simulink model "transmitter"  (R2020b)
settings: Solver=FixedStepDiscrete  StartTime=0.0  StopTime=100000  RelTol=1e-3
undefined symbols (not defined in the file): message
libraries: hdlsllib x24, simulink x11, dspmlti4 x2, whdlio x1
(part 1 of 2)
settings Model: DataTypeOverride=Off  Creator=wardo  LastModifiedBy=wardo
settings DataIOCC: LimitDataPoints=on  SaveOutput=off  SaveTime=off
settings OptimizationCC: BlockReduction=off  ConditionallyExecuteInputs=off  DefaultParameterBehavior=Inlined  LifeSpan=inf
settings DebuggingCC: AlgebraicLoopMsg=error  SingleTaskRateTransMsg=error  AllowSymbolicDim=off  StrictBusMsg=ErrorOnBusTreatedAsVector  SFUnexpectedBacktrackingDiag=warning  SFNoUnconditionalDefaultTransitionDiag=warning  SFExecutionAtInitializationDiag=none  ArithmeticOperatorsInVariantConditions=warning
settings HardwareCC: ProdBitPerPointer=32  ProdBitPerSizeT=32  ProdBitPerPtrDiffT=32  ProdLargestAtomicFloat=None  ProdIntDivRoundTo=Undefined  ProdEndianess=Unspecified  ProdWordSize=32  ProdHWDeviceType=ASIC/FPGA->ASIC/FPGA  ProdEqTarget=off
settings SFSimCC: SimUseLocalCustomCode=off  CustomCodeUndefinedFunction=UseInterfaceOnly
settings RTWCC: RTWUseLocalCustomCode=off
settings CodeAppCC: StateflowObjectComments=on
settings GRTTargetCC: TargetLangStandard=C89/C90 (ANSI)
settings ConfigComp: CovScope=ReferencedModels  CovMetricSettings=dw  CovSaveCumulativeToWorkspaceVar=on  CovSaveSingleToWorkspaceVar=on  CovExternalEMLEnable=off  CovSFcnEnable=off

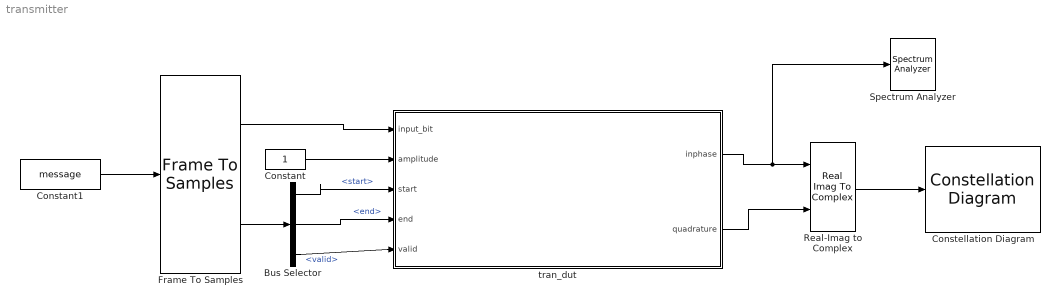
== system transmitter ==
  Bus Selector : BusSelector  OutputSignals=start,end,valid
  Constant : Constant  OutDataTypeStr=uint8  SampleTime=-1
  Constant1 : Constant  Value=message  OutDataTypeStr=fixdt(0,1,0)  SampleTime=100000
  Constellation Diagram : ConstellationDiagram
  Frame To Samples : whdlio/Frame To Samples  InterSampleIdleCycles=0  InterFrameIdleCycles=0  OutputSize=1  InterleaveSamples=off
      settings: SourceProductBaseCode=LH
  Real-Imag to Complex : RealImagToComplex
  Spectrum Analyzer : SpectrumAnalyzer
  tran_dut : Subsystem
  wires:
  Frame To Samples/1 -> tran_dut/1(input_bit)
  Constant/1 -> tran_dut/2(amplitude)
  Constant1/1 -> Frame To Samples/1
  Real-Imag to Complex/1 -> Constellation Diagram/1
  tran_dut/1(inphase) -> Spectrum Analyzer/1, Real-Imag to Complex/1
  tran_dut/2(quadrature) -> Real-Imag to Complex/2
  Frame To Samples/2 -> Bus Selector/1
  Bus Selector/1 -> tran_dut/3(start)  "<start>"
  Bus Selector/2 -> tran_dut/4(end)  "<end>"
  Bus Selector/3 -> tran_dut/5(valid)  "<valid>"

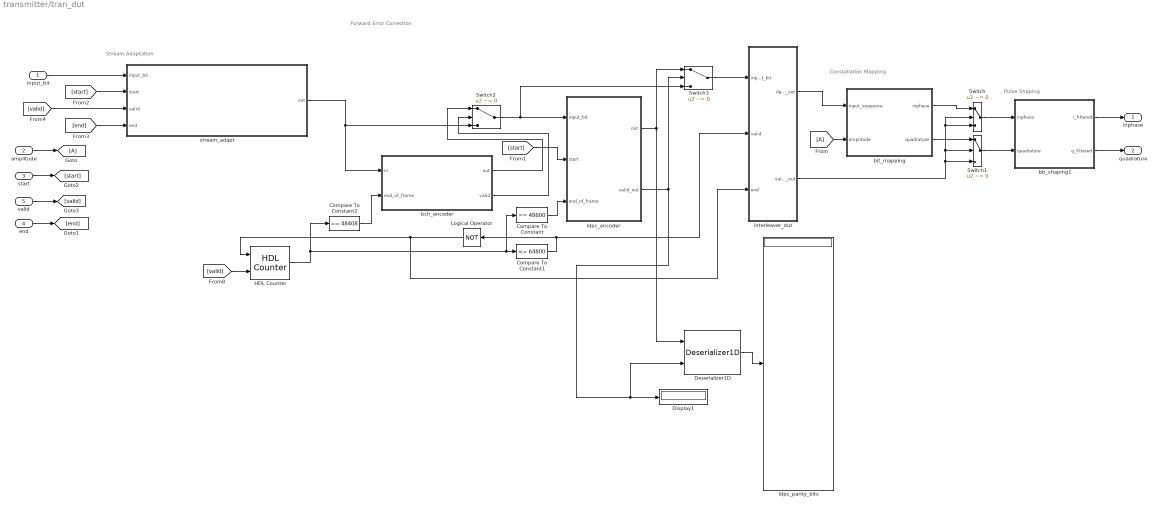
== system transmitter/tran_dut ==
  note: Pulse Shaping
  note: Constellation Mapping
  note: Forward Error Correction
  note: Stream Adaptation
  input_bit : Inport
  amplitude : Inport  Port=2
  start : Inport  Port=3
  end : Inport  Port=4
  valid : Inport  Port=5
  Compare To Constant : simulink/Logic and Bit Operations/Compare To Constant  relop===  const=48600  OutDataTypeStr=boolean
  Compare To Constant1 : simulink/Logic and Bit Operations/Compare To Constant  relop=<=  const=64800  OutDataTypeStr=boolean
  Compare To Constant2 : simulink/Logic and Bit Operations/Compare To Constant  relop===  const=48408  OutDataTypeStr=boolean
  Deserializer1D : hdlsllib/HDL Operations/Deserializer1D  Ratio=16200  IdleCycles=0  InitialCondition=0  startIn=off  validIn=on  validOut=off  inputDataDimensions=-1  inputSampleTime=-1  inputSignalType=auto
      settings: SourceProductBaseCode=SL
  Display1 : Display
  HDL Counter : hdlsllib/Sources/HDL Counter  CountType=Count limited  CountInit=0  CountStep=1  CountMax=64800  CountFromType=Initial value  CountFrom=0  CountResetPort=on  CountLoadPort=off  CountEnbPort=on  CountDirPort=off  CountDataType=Unsigned  CountWordLen=16  CountFracLen=0  CountSampTime=1
  Logical Operator : Logic  Operator=NOT  IconShape=distinctive  AllPortsSameDT=off  OutDataTypeStr=boolean
  Switch : Switch  Criteria=u2 ~= 0  OutDataTypeStr=Inherit: Inherit via back propagation
  Switch1 : Switch  Criteria=u2 ~= 0  OutDataTypeStr=Inherit: Inherit via back propagation
  Switch2 : Switch  Criteria=u2 ~= 0  OutDataTypeStr=boolean
  Switch3 : Switch  Criteria=u2 ~= 0  OutDataTypeStr=boolean
  bb_shaping1 : Subsystem
  bch_encoder : Subsystem
  bit_mapping : Subsystem
  interleaver_dut : Subsystem
  ldpc_encoder : Subsystem
  ldpc_parity_bits : Display
  stream_adapt : Subsystem
  inphase : Outport  VectorParamsAs1DForOutWhenUnconnected=off
  quadrature : Outport  Port=2  VectorParamsAs1DForOutWhenUnconnected=off
  wires:
  bb_shaping1/1(i_filtered) -> inphase/1
  bb_shaping1/2(q_filtered) -> quadrature/1
  bit_mapping/2(quadrature) -> Switch1/1
  bit_mapping/1(inphase) -> Switch/1
  interleaver_dut/2(valid_out) -> Switch1/2, Switch/2, Switch/3, Switch1/3
  Switch/1 -> bb_shaping1/1(inphase)
  Switch1/1 -> bb_shaping1/2(quadrature)
  ldpc_encoder/1(out) -> Deserializer1D/1, Switch3/1
  Deserializer1D/1 -> ldpc_parity_bits/1
  ldpc_encoder/2(valid_out) -> Deserializer1D/2, Display1/1, Switch3/2
  stream_adapt/1(out) -> Switch2/3, bch_encoder/1(in)
  Switch2/1 -> ldpc_encoder/1(input_bit), Switch3/3
  bch_encoder/2(valid) -> Switch2/2
  amplitude/1 -> [A]
  [A] -> bit_mapping/2(amplitude)
  end/1 -> [end]
  bch_encoder/1(out) -> Switch2/1
  start/1 -> [start]
  [start] -> stream_adapt/2(start)
  input_bit/1 -> stream_adapt/1(input_bit)
  [end] -> stream_adapt/4(end)
  valid/1 -> [valid]
  [valid] -> stream_adapt/3(valid)
  Compare To Constant2/1 -> bch_encoder/2(end_of_frame)
  Switch3/1 -> interleaver_dut/1(input_bit)
  [start] -> ldpc_encoder/2(start)
  HDL Counter/1 -> Compare To Constant2/1, Compare To Constant/1, Compare To Constant1/1
  Compare To Constant/1 -> ldpc_encoder/3(end_of_frame)
  [valid] -> HDL Counter/2
  Compare To Constant1/1 -> interleaver_dut/2(valid), Logical Operator/1
  Logical Operator/1 -> interleaver_dut/3(end), HDL Counter/1
  interleaver_dut/1(data_out) -> bit_mapping/1(input_sequence)

== system transmitter/tran_dut/bb_shaping1 ==
  inphase : Inport
  quadrature : Inport  Port=2
  FIR Interpolation : dspmlti4/FIR Interpolation  FilterSource=Dialog parameters  PrivateCoeffs=0  h=[-0.00599670410156250,-0.00514221191406250,-0.00289916992187500,0.000442504882812500,0.00431823730468750,0.00794982910156250,0.0104980468750000,0.0112304687500000,0.00967407226562500,0.00578308105468750,0,-0.00680541992187500,-0.0134124755859375,-0.0184326171875000,-0.0205841064453125,-0.0189819335937500,-0.0133361816406250,-0.00410461425781250,0.00752258300781250,0.0196380615234375,0.0300140380859375,0.0363464355468750,0.0367584228515625,0.0301208496093750,0.0164794921875000,-0.00291442871093750,-0.0254821777343750,-0.0476837158203125,-0.0653228759765625,-0.0742187500000000,-0.0707244873046875,-0.0524291992187500,-0.0185852050781250,0.0296783447265625,0.0892028808593750,0.155227661132813,0.221755981445313,0.282333374023438,0.330810546875000,0.362121582031250,0.372940063476563,0.362121582031250,0.330810546875000,0.282333374023438,0.221755981445313,0.155227661132813,0.0892028808593750,0.0296783447265625,-0.0185852050781250,-0.0524291992187500,-0.0707244873046875,-0.0742187500000000,-0.0653228759765625,-0.0476837158203125,-0.0254821777343750,-0.00291442871093750,0.0164794921875000,0.0301208496093750,0.0367584228515625,0.0363464355468750,0.0300140380859375,0.0196380615234375,0.00752258300781250,-0.00410461425781250,-0.0133361816406250,-0.0189819335937500,-0.0205841064453125,-0.0184326171875000,-0.0134124755859375,-0.00680541992187500,0,0.00578308105468750,0.00967407226562500,0.0112304687500000,0.0104980468750000,0.00794982910156250,0.00431823730468750,0.000442504882812500,-0.00289916992187500,-0.00514221191406250,-0.00599670410156250]  L=8  FilterObject=FINTERP  framing=Allow multirate processing  outputBufInitCond=0  roundingMode=Floor  overflowMode=off  firstCoeffMode=Specify word length  firstCoeffWordLength=16  firstCoeffFracLength=15  firstCoeffDataTypeStr=fixdt(1,16)  firstCoeffMin=[]  firstCoeffMax=[]  firstCoeffLastDataTypeStr=fixdt(1,16)  outputDataTypeStr=Inherit: Same as accumulator  outputMin=[]  outputMax=[]  outputLastDataTypeStr=Inherit: Same as accumulator
      settings: SourceProductName=DSP System Toolbox
  FIR Interpolation1 : dspmlti4/FIR Interpolation  FilterSource=Dialog parameters  PrivateCoeffs=0  h=[-0.00599670410156250,-0.00514221191406250,-0.00289916992187500,0.000442504882812500,0.00431823730468750,0.00794982910156250,0.0104980468750000,0.0112304687500000,0.00967407226562500,0.00578308105468750,0,-0.00680541992187500,-0.0134124755859375,-0.0184326171875000,-0.0205841064453125,-0.0189819335937500,-0.0133361816406250,-0.00410461425781250,0.00752258300781250,0.0196380615234375,0.0300140380859375,0.0363464355468750,0.0367584228515625,0.0301208496093750,0.0164794921875000,-0.00291442871093750,-0.0254821777343750,-0.0476837158203125,-0.0653228759765625,-0.0742187500000000,-0.0707244873046875,-0.0524291992187500,-0.0185852050781250,0.0296783447265625,0.0892028808593750,0.155227661132813,0.221755981445313,0.282333374023438,0.330810546875000,0.362121582031250,0.372940063476563,0.362121582031250,0.330810546875000,0.282333374023438,0.221755981445313,0.155227661132813,0.0892028808593750,0.0296783447265625,-0.0185852050781250,-0.0524291992187500,-0.0707244873046875,-0.0742187500000000,-0.0653228759765625,-0.0476837158203125,-0.0254821777343750,-0.00291442871093750,0.0164794921875000,0.0301208496093750,0.0367584228515625,0.0363464355468750,0.0300140380859375,0.0196380615234375,0.00752258300781250,-0.00410461425781250,-0.0133361816406250,-0.0189819335937500,-0.0205841064453125,-0.0184326171875000,-0.0134124755859375,-0.00680541992187500,0,0.00578308105468750,0.00967407226562500,0.0112304687500000,0.0104980468750000,0.00794982910156250,0.00431823730468750,0.000442504882812500,-0.00289916992187500,-0.00514221191406250,-0.00599670410156250]  L=8  FilterObject=FINTERP  framing=Allow multirate processing  outputBufInitCond=0  roundingMode=Floor  overflowMode=off  firstCoeffMode=Specify word length  firstCoeffWordLength=16  firstCoeffFracLength=15  firstCoeffDataTypeStr=fixdt(1,16)  firstCoeffMin=[]  firstCoeffMax=[]  firstCoeffLastDataTypeStr=fixdt(1,16)  outputDataTypeStr=Inherit: Same as accumulator  outputMin=[]  outputMax=[]  outputLastDataTypeStr=Inherit: Same as accumulator
      settings: SourceProductName=DSP System Toolbox
  i_filtered : Outport  VectorParamsAs1DForOutWhenUnconnected=off
  q_filtered : Outport  Port=2  VectorParamsAs1DForOutWhenUnconnected=off
  wires:
  inphase/1 -> FIR Interpolation/1
  FIR Interpolation/1 -> i_filtered/1
  FIR Interpolation1/1 -> q_filtered/1
  quadrature/1 -> FIR Interpolation1/1

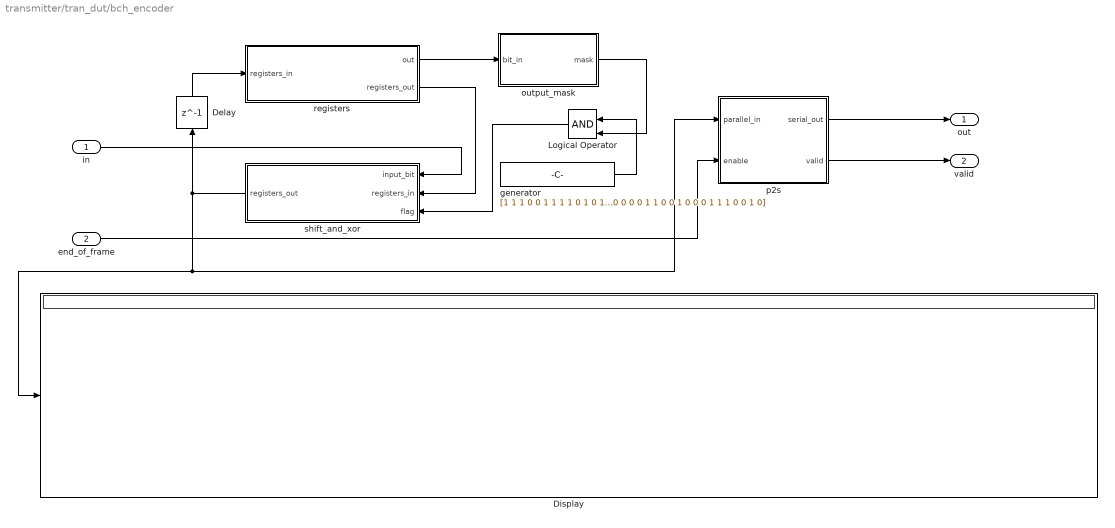
== system transmitter/tran_dut/bch_encoder ==
  in : Inport
  end_of_frame : Inport  Port=2
  Delay : Delay  DelayLength=1
  Display : Display
  Logical Operator : Logic  IconShape=distinctive  AllPortsSameDT=off  OutDataTypeStr=fixdt(0, 1, 0)
  generator : Constant  Value=|  OutDataTypeStr=fixdt(0, 1, 0)  SampleTime=-1
      | [1
      | 1
      | 1
      | 0
      | 0
      | 1
      | 1
      | 1
      | 1
      | 0
      | 1
      | 0
      | 1
      | 0
      | 1
      | 0
      | 0
      | 1
      | 0
      | 0
      | 0
      | 0
      | 0
      | 0
      | 0
      | 1
      | 1
      | 0
      | 0
      | 1
      | 1
      | 0
      | 1
      | 1
      | 1
      | 0
      | 1
      | 1
      | 1
      | 1
      | 1
      | 0
      | 1
      | 0
      | 0
      | 0
      | 0
      | 1
      | 1
      | 1
      | 1
      | 0
      | 0
      | 0
      | 1
      | 0
      | 1
      | 1
      | 0
      | 0
      | 0
      | 0
      | 0
      | 0
      | 1
      | 0
      | 0
      | 1
      | 0
      | 0
      | 0
      | 1
      | 0
      | 0
      | 0
      | 1
      | 0
      | 0
      | 0
      | 0
      | 1
      | 0
      | 1
      | 0
      | 1
      | 1
      | 0
      | 0
      | 0
      | 0
      | 1
      | 1
      | 1
      | 0
      | 1
      | 1
      | 0
      | 0
      | 0
      | 1
      | 1
      | 0
      | 1
      | 1
      | 0
      | 0
      | 1
      | 1
      | 0
      | 1
      | 0
      | 0
      | 1
      | 1
      | 1
      | 1
      | 0
      | 0
      | 1
      | 1
      | 0
      | 0
      | 0
      | 0
      | 1
      | 0
      | 1
      | 0
      | 0
      | 0
      | 1
      | 1
      | 1
      | 0
      | 0
      | 0
      | 1
      | 0
      | 0
      | 0
      | 1
      | 0
      | 1
      | 0
      | 0
      | 0
      | 1
      | 1
      | 1
      | 0
      | 1
      | 0
      | 0
      | 0
      | 1
      | 0
      | 0
      | 0
      | 0
      | 1
      | 1
      | 1
      | 0
      | 0
      | 0
      | 0
      | 0
      | 1
      | 0
      | 1
      | 1
      | 1
      | 0
      | 0
      | 0
      | 0
      | 0
      | 1
      | 1
      | 0
      | 0
      | 1
      | 0
      | 0
      | 0
      | 1
      | 1
      | 1
      | 0
      | 0
      | 1
      | 0]
  output_mask : MATLAB Function  TreatAsAtomicUnit=on
  p2s : MATLAB Function  TreatAsAtomicUnit=on  mask{input_length=192}
  registers : MATLAB Function  TreatAsAtomicUnit=on
  shift_and_xor : MATLAB Function  TreatAsAtomicUnit=on
  out : Outport  VectorParamsAs1DForOutWhenUnconnected=off
  valid : Outport  Port=2  VectorParamsAs1DForOutWhenUnconnected=off
  wires:
  registers/1(out) -> output_mask/1(bit_in)
  output_mask/1(mask) -> Logical Operator/2
  generator/1 -> Logical Operator/1
  Logical Operator/1 -> shift_and_xor/3(flag)
  registers/2(registers_out) -> shift_and_xor/2(registers_in)
  shift_and_xor/1(registers_out) -> p2s/1(parallel_in), Display/1, Delay/1
  in/1 -> shift_and_xor/1(input_bit)
  Delay/1 -> registers/1(registers_in)
  end_of_frame/1 -> p2s/2(enable)
  p2s/1(serial_out) -> out/1
  p2s/2(valid) -> valid/1

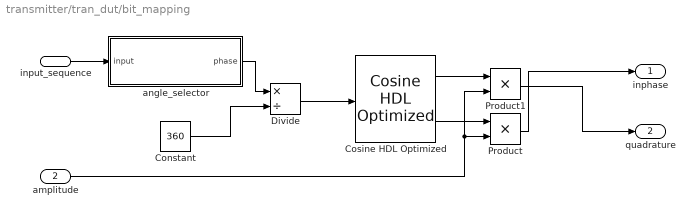
== system transmitter/tran_dut/bit_mapping ==
  input_sequence : Inport
  amplitude : Inport  Port=2
  Constant : Constant  Value=360  OutDataTypeStr=fixdt(0,9,0)  SampleTime=-1
  Cosine HDL Optimized : hdlsllib/Lookup Tables/Cosine HDL Optimized  OutputFormula=sin(2*pi*u) and cos(2*pi*u)  NumDataPoints=32  TableDataTypeStr=fixdt(1,16,15)  SimulateLUTROMDelay=off
      settings: SourceProductBaseCode=SL
  Divide : Product  Inputs=*/  OutMin=0  OutMax=1  OutDataTypeStr=fixdt(1,16,14)  RndMeth=Zero  SaturateOnIntegerOverflow=on
  Product : Product
  Product1 : Product
  angle_selector : MATLAB Function  TreatAsAtomicUnit=on
  inphase : Outport  VectorParamsAs1DForOutWhenUnconnected=off
  quadrature : Outport  Port=2  VectorParamsAs1DForOutWhenUnconnected=off
  wires:
  Product/1 -> inphase/1
  Product1/1 -> quadrature/1
  input_sequence/1 -> angle_selector/1(input)
  amplitude/1 -> Product1/2, Product/2
  Cosine HDL Optimized/2 -> Product/1
  Cosine HDL Optimized/1 -> Product1/1
  Divide/1 -> Cosine HDL Optimized/1
  angle_selector/1(phase) -> Divide/1
  Constant/1 -> Divide/2

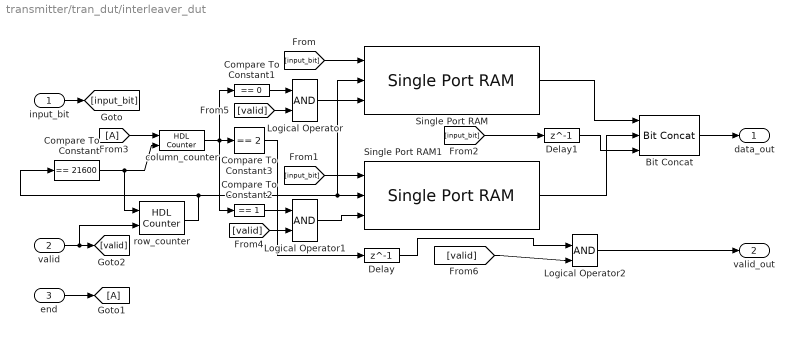
== system transmitter/tran_dut/interleaver_dut ==
  input_bit : Inport
  valid : Inport  Port=2
  end : Inport  Port=3
  Bit Concat : hdlsllib/Logic and Bit Operations/Bit Concat  numInputs=3
  Compare To Constant : simulink/Logic and Bit Operations/Compare To Constant  relop===  const=21600  OutDataTypeStr=boolean
  Compare To Constant1 : simulink/Logic and Bit Operations/Compare To Constant  relop===  const=0  OutDataTypeStr=boolean
  Compare To Constant2 : simulink/Logic and Bit Operations/Compare To Constant  relop===  const=1  OutDataTypeStr=boolean
  Compare To Constant3 : simulink/Logic and Bit Operations/Compare To Constant  relop===  const=2  OutDataTypeStr=boolean
  Delay : Delay  DelayLength=1
  Delay1 : Delay  DelayLength=1
  Logical Operator : Logic  IconShape=distinctive  AllPortsSameDT=off  OutDataTypeStr=boolean
  Logical Operator1 : Logic  IconShape=distinctive  AllPortsSameDT=off  OutDataTypeStr=boolean
  Logical Operator2 : Logic  IconShape=distinctive  AllPortsSameDT=off  OutDataTypeStr=boolean
  Single Port RAM : hdlsllib/HDL RAMs/Single Port RAM  ram_size=15  dout_type=New data
      settings: SourceProductBaseCode=SL
  Single Port RAM1 : hdlsllib/HDL RAMs/Single Port RAM  ram_size=15  dout_type=New data
      settings: SourceProductBaseCode=SL
  column_counter : hdlsllib/Sources/HDL Counter  CountType=Count limited  CountInit=0  CountStep=1  CountMax=2  CountFromType=Initial value  CountFrom=0  CountResetPort=on  CountLoadPort=off  CountEnbPort=on  CountDirPort=off  CountDataType=Unsigned  CountWordLen=3  CountFracLen=0  CountSampTime=1
  row_counter : hdlsllib/Sources/HDL Counter  CountType=Count limited  CountInit=1  CountStep=1  CountMax=21600  CountFromType=Initial value  CountFrom=1  CountResetPort=on  CountLoadPort=off  CountEnbPort=on  CountDirPort=off  CountDataType=Unsigned  CountWordLen=15  CountFracLen=0  CountSampTime=1
  data_out : Outport  VectorParamsAs1DForOutWhenUnconnected=off
  valid_out : Outport  Port=2  VectorParamsAs1DForOutWhenUnconnected=off
  wires:
  Bit Concat/1 -> data_out/1
  Logical Operator2/1 -> valid_out/1
  row_counter/1 -> Single Port RAM/2, Single Port RAM1/2, Compare To Constant/1
  Compare To Constant/1 -> column_counter/2, row_counter/1
  input_bit/1 -> [input_bit]
  [input_bit] -> Single Port RAM/1
  [input_bit] -> Single Port RAM1/1
  Compare To Constant1/1 -> Logical Operator/1
  column_counter/1 -> Compare To Constant1/1, Compare To Constant3/1, Compare To Constant2/1
  Logical Operator/1 -> Single Port RAM/3
  Logical Operator1/1 -> Single Port RAM1/3
  Compare To Constant2/1 -> Logical Operator1/1
  Single Port RAM1/1 -> Bit Concat/2
  Single Port RAM/1 -> Bit Concat/1
  Compare To Constant3/1 -> Delay/1
  [input_bit] -> Delay1/1
  end/1 -> [A]
  [A] -> column_counter/1
  valid/1 -> row_counter/2, [valid]
  [valid] -> Logical Operator2/2
  [valid] -> Logical Operator/2
  [valid] -> Logical Operator1/2
  Delay/1 -> Logical Operator2/1
  Delay1/1 -> Bit Concat/3

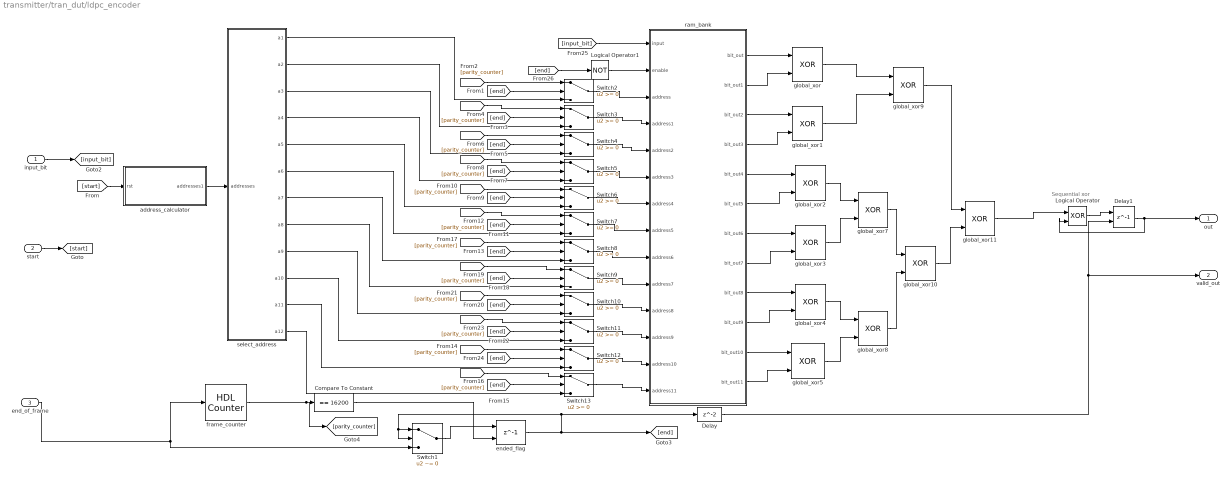
== system transmitter/tran_dut/ldpc_encoder ==
  note: Sequential xor
  input_bit : Inport
  start : Inport  Port=2
  end_of_frame : Inport  Port=3
  Compare To Constant : simulink/Logic and Bit Operations/Compare To Constant  relop===  const=16200  OutDataTypeStr=boolean
  Delay : Delay
  Delay1 : Delay  DelayLength=1  ShowEnablePort=on
      settings: InputPortMap=u0,e6
  Logical Operator : Logic  Operator=XOR  IconShape=distinctive  AllPortsSameDT=off  OutDataTypeStr=fixdt(0,1, 0)
  Logical Operator1 : Logic  Operator=NOT  IconShape=distinctive  AllPortsSameDT=off  OutDataTypeStr=boolean
  Switch1 : Switch  Criteria=u2 ~= 0  OutDataTypeStr=boolean
  Switch{2..13} (12 alike) : Switch
  address_calculator : Subsystem
  ended_flag : Delay  DelayLength=1  ExternalReset=Level
      settings: InputPortMap=u0,r5
  frame_counter : hdlsllib/Sources/HDL Counter  CountType=Count limited  CountInit=0  CountStep=1  CountMax=16200  CountFromType=Initial value  CountFrom=0  CountResetPort=on  CountLoadPort=off  CountEnbPort=off  CountDirPort=off  CountDataType=Unsigned  CountWordLen=14  CountFracLen=0  CountSampTime=1
  global_xor{,1..5,7..11} (11 alike) : Logic  Operator=XOR  IconShape=distinctive  AllPortsSameDT=off  OutDataTypeStr=boolean
  ram_bank : Subsystem
  select_address : MATLAB Function  TreatAsAtomicUnit=on
  out : Outport  VectorParamsAs1DForOutWhenUnconnected=off
  valid_out : Outport  Port=2  VectorParamsAs1DForOutWhenUnconnected=off
  wires:
  input_bit/1 -> [input_bit]
  start/1 -> [start]
  address_calculator/1(addresses1) -> select_address/1(addresses)
  [start] -> address_calculator/1(rst)
  Logical Operator/1 -> Delay1/1
  Delay1/1 -> out/1, Logical Operator/2
  Compare To Constant/1 -> ended_flag/2
  Switch1/1 -> ended_flag/1
  frame_counter/1 -> [parity_counter], Compare To Constant/1
  ram_bank/1(bit_out) -> global_xor/1
  [end] -> Switch2/2
  select_address/1(a1) -> Switch2/3
  [parity_counter] -> Switch2/1
  Switch3/1 -> ram_bank/4(address1)
  [parity_counter] -> Switch3/1
  [end] -> Switch3/2
  select_address/2(a2) -> Switch3/3
  [end] -> Switch5/2
  select_address/3(a3) -> Switch4/3
  [parity_counter] -> Switch5/1
  [end] -> Switch4/2
  select_address/4(a4) -> Switch5/3
  [parity_counter] -> Switch4/1
  [parity_counter] -> Switch7/1
  [end] -> Switch6/2
  [parity_counter] -> Switch6/1
  [end] -> Switch7/2
  select_address/5(a5) -> Switch6/3
  select_address/6(a6) -> Switch7/3
  [end] -> Switch10/2
  [end] -> Switch9/2
  [end] -> Switch11/2
  [parity_counter] -> Switch13/1
  select_address/10(a10) -> Switch11/3
  select_address/11(a11) -> Switch12/3
  [parity_counter] -> Switch11/1
  [end] -> Switch8/2
  [end] -> Switch13/2
  select_address/8(a8) -> Switch9/3
  select_address/9(a9) -> Switch10/3
  [end] -> Switch12/2
  select_address/12(a12) -> Switch13/3
  [parity_counter] -> Switch12/1
  [parity_counter] -> Switch10/1
  [parity_counter] -> Switch9/1
  select_address/7(a7) -> Switch8/3
  [parity_counter] -> Switch8/1
  [input_bit] -> ram_bank/1(input)
  Switch2/1 -> ram_bank/3(address)
  Logical Operator1/1 -> ram_bank/2(enable)
  ram_bank/2(bit_out1) -> global_xor/2
  ram_bank/3(bit_out2) -> global_xor1/1
  ram_bank/4(bit_out3) -> global_xor1/2
  ram_bank/6(bit_out5) -> global_xor2/2
  ram_bank/8(bit_out7) -> global_xor3/2
  ram_bank/9(bit_out8) -> global_xor4/1
  ram_bank/10(bit_out9) -> global_xor4/2
  ram_bank/11(bit_out10) -> global_xor5/1
  ram_bank/12(bit_out11) -> global_xor5/2
  Switch4/1 -> ram_bank/5(address2)
  Switch5/1 -> ram_bank/6(address3)
  Switch6/1 -> ram_bank/7(address4)
  Switch7/1 -> ram_bank/8(address5)
  Switch8/1 -> ram_bank/9(address6)
  Switch9/1 -> ram_bank/10(address7)
  Switch10/1 -> ram_bank/11(address8)
  Switch11/1 -> ram_bank/12(address9)
  Switch12/1 -> ram_bank/13(address10)
  Switch13/1 -> ram_bank/14(address11)
  ram_bank/7(bit_out6) -> global_xor3/1
  ram_bank/5(bit_out4) -> global_xor2/1
  global_xor11/1 -> Logical Operator/1
  global_xor9/1 -> global_xor11/1
  global_xor10/1 -> global_xor11/2
  global_xor8/1 -> global_xor10/2
  global_xor7/1 -> global_xor10/1
  global_xor/1 -> global_xor9/1
  global_xor1/1 -> global_xor9/2
  global_xor2/1 -> global_xor7/1
  global_xor3/1 -> global_xor7/2
  global_xor4/1 -> global_xor8/1
  global_xor5/1 -> global_xor8/2
  ended_flag/1 -> [end], Switch1/2, Switch1/1, Delay/1
  [end] -> Logical Operator1/1
  end_of_frame/1 -> frame_counter/1, Switch1/3
  Delay/1 -> valid_out/1, Delay1/2

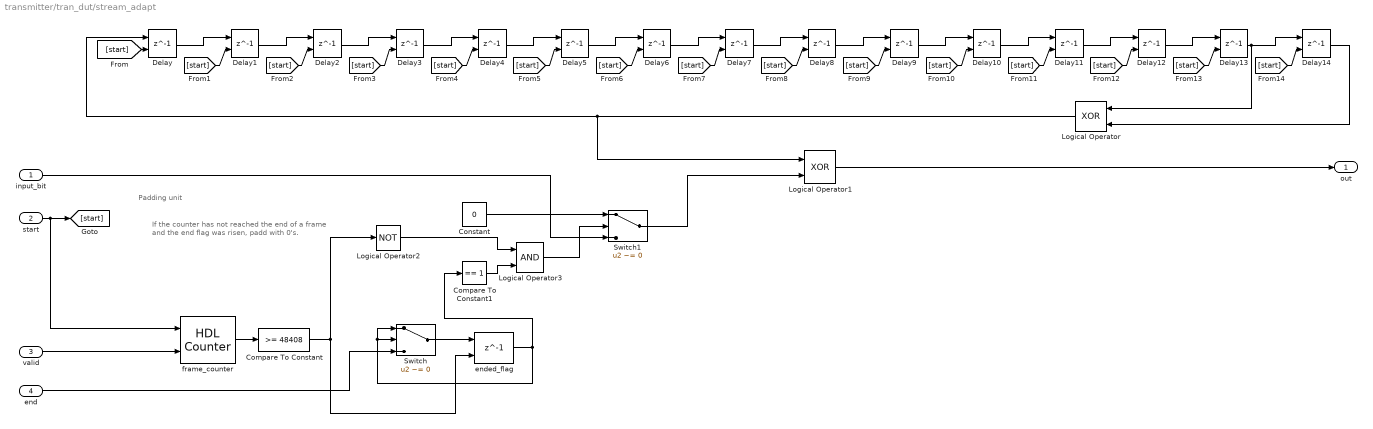
== system transmitter/tran_dut/stream_adapt ==
  note: Padding unit
  note: If the counter has not reached the end of a frame and the end flag was risen,
      | padd with 0's.
  input_bit : Inport
  start : Inport  Port=2
  valid : Inport  Port=3
  end : Inport  Port=4
  Compare To Constant : simulink/Logic and Bit Operations/Compare To Constant  relop=>=  const=48408  OutDataTypeStr=boolean
  Compare To Constant1 : simulink/Logic and Bit Operations/Compare To Constant  relop===  const=1  OutDataTypeStr=boolean
  Constant : Constant  Value=0  OutDataTypeStr=fixdt(0,1)  SampleTime=-1
  Delay{,3,5,7} (4 alike) : Delay  DelayLength=1  InitialCondition=1  ExternalReset=Level
      settings: InputPortMap=u0,r5
  Delay{1..2,4,6,8..14} (11 alike) : Delay  DelayLength=1  ExternalReset=Level
      settings: InputPortMap=u0,r5
  Logical Operator : Logic  Operator=XOR  IconShape=distinctive  AllPortsSameDT=off  OutDataTypeStr=boolean
  Logical Operator1 : Logic  Operator=XOR  IconShape=distinctive  AllPortsSameDT=off  OutDataTypeStr=boolean
  Logical Operator2 : Logic  Operator=NOT  IconShape=distinctive  AllPortsSameDT=off  OutDataTypeStr=boolean
  Logical Operator3 : Logic  IconShape=distinctive  AllPortsSameDT=off  OutDataTypeStr=boolean
  Switch : Switch  Criteria=u2 ~= 0  OutDataTypeStr=boolean
  Switch1 : Switch  Criteria=u2 ~= 0
  ended_flag : Delay  DelayLength=1  ExternalReset=Level
      settings: InputPortMap=u0,r5
  frame_counter : hdlsllib/Sources/HDL Counter  CountType=Count limited  CountInit=0  CountStep=1  CountMax=48408  CountFromType=Initial value  CountFrom=0  CountResetPort=on  CountLoadPort=off  CountEnbPort=on  CountDirPort=off  CountDataType=Unsigned  CountWordLen=16  CountFracLen=0  CountSampTime=1
  out : Outport  VectorParamsAs1DForOutWhenUnconnected=off
  wires:
  Delay/1 -> Delay1/1
  Logical Operator/1 -> Delay/1, Logical Operator1/1
  Logical Operator1/1 -> out/1
  start/1 -> frame_counter/1, [start]
  [start] -> Delay/2
  [start] -> Delay1/2
  Delay1/1 -> Delay2/1
  [start] -> Delay2/2
  Delay2/1 -> Delay3/1
  [start] -> Delay3/2
  Delay3/1 -> Delay4/1
  [start] -> Delay4/2
  Delay4/1 -> Delay5/1
  [start] -> Delay5/2
  Delay5/1 -> Delay6/1
  [start] -> Delay6/2
  Delay6/1 -> Delay7/1
  [start] -> Delay7/2
  Delay7/1 -> Delay8/1
  [start] -> Delay8/2
  Delay8/1 -> Delay9/1
  [start] -> Delay9/2
  Delay9/1 -> Delay10/1
  [start] -> Delay10/2
  Delay10/1 -> Delay11/1
  [start] -> Delay11/2
  Delay11/1 -> Delay12/1
  [start] -> Delay12/2
  Delay12/1 -> Delay13/1
  [start] -> Delay13/2
  Delay13/1 -> Logical Operator/1, Delay14/1
  [start] -> Delay14/2
  Delay14/1 -> Logical Operator/2
  valid/1 -> frame_counter/2
  frame_counter/1 -> Compare To Constant/1
  Compare To Constant/1 -> ended_flag/2, Logical Operator2/1
  Switch/1 -> ended_flag/1
  end/1 -> Switch/3
  ended_flag/1 -> Switch/1, Switch/2, Compare To Constant1/1
  Compare To Constant1/1 -> Logical Operator3/2
  Logical Operator3/1 -> Switch1/2
  Logical Operator2/1 -> Logical Operator3/1
  Switch1/1 -> Logical Operator1/2
  input_bit/1 -> Switch1/3
  Constant/1 -> Switch1/1

== system transmitter/tran_dut/ldpc_encoder/address_calculator ==
  rst : Inport
  addresses : MATLAB Function  TreatAsAtomicUnit=on  mask{bit_addresses=uint16([[0 6385 7901 14611 13389 11200 3252 5243 2504 2722 821 7374]; [1 11359 2698 357 13824 12772 7244 6752 15310 852 2001 11417]; [2 7862 7977 6321 13612 12197 14449 15137 13860 1708 6399 13444]; [3 1560 11804 6975 13292 3646 3812 8772 7306 5795 14327 7866]; [4 7626 11407 14599 9689 1628 2113 10809 9283 1230 15241 4870]; [5 1610 5699 15876 9446 12515 1400 6303 5411 14181 13925 7358]; [6 4059 8836 3405 7853 7992 15336 5970 10368 10278 9675 4651]; [7 4441 3963 9153 2109 12683 7459 12030 12221 629 15212 406]; [8 6007 8411 5771 3497 543 14202 875 9186 6235 13908 3563]; [9 3232 6625 4795 546 9781 2071 7312 3399 7250 4932 12652]; [10 8820 10088 11090 7069 6585 13134 10158 7183 488 7455 9238]; [11 1903 10818 119 215 7558 11046 10615 11545 14784 7961 15619]; [12 3655 8736 4917 15874 5129 2134 15944 14768 7150 2692 1469]; [13 8316 3820 505 8923 6757 806 7957 4216 15589 13244 2622]; [14 14463 4852 15733 3041 11193 12860 13673 8152 6551 15108 8758]; [15 3149 11981 16200 16200 16200 16200 16200 16200 16200 16200 16200]; [16 13416 6906 16200 16200 16200 16200 16200 16200 16200 16200 16200]; [17 13098 13352 16200 16200 16200 16200 16200 16200 16200 16200 16200]; [18 2009 14460 16200 16200 16200 16200 16200 16200 16200 16200 16200]; [19 7207 4314 16200 16200 16200 16200 16200 16200 16200 16200 16200]; [20 3312 3945 16200 16200 16200 16200 16200 16200 16200 16200 16200]; [21 4418 6248 16200 16200 16200 16200 16200 16200 16200 16200 16200]; [22 2669 13975 16200 16200 16200 16200 16200 16200 16200 16200 16200]; [23 7571 9023 16200 16200 16200 16200 16200 16200 16200 16200 16200]; [24 14172 2967 16200 16200 16200 16200 16200 16200 16200 16200 16200]; [25 7271 7138 16200 16200 16200 16200 16200 16200 16200 16200 16200]; [26 6135 13670 16200 16200 16200 16200 16200 16200 16200 16200 16200]; [27 7490 14559 16200 16200 16200 16200 16200 16200 16200 16200 16200]; [28 8657 2466 16200 16200 16200 16200 16200 16200 16200 16200 16200]; [29 8599 12834 16200 16200 16200 16200 16200 16200 16200 16200 16200]; [30 3470 3152 16200 16200 16200 16200 16200 16200 16200 16200 16200]; [31 13917 4365 16200 16200 16200 16200 16200 16200 16200 16200 16200]; [32 6024 13730 16200 16200 16200 16200 16200 16200 16200 16200 16200]; [33 10973 14182 16200 16200 16200 16200 16200 16200 16200 16200 16200]; [34 2464 13167 16200 16200 16200 16200 16200 16200 16200 16200 16200]; [35 5281 15049 16200 16200 16200 16200 16200 16200 16200 16200 16200]; [36 1103 1849 16200 16200 16200 16200 16200 16200 16200 16200 16200]; [37 2058 1069 16200 16200 16200 16200 16200 16200 16200 16200 16200]; [38 9654 6095 16200 16200 16200 16200 16200 16200 16200 16200 16200]; [39 14311 7667 16200 16200 16200 16200 16200 16200 16200 16200 16200]; [40 15617 8146 16200 16200 16200 16200 16200 16200 16200 16200 16200]; [41 4588 11218 16200 16200 16200 16200 16200 16200 16200 16200 16200]; [42 13660 6243 16200 16200 16200 16200 16200 16200 16200 16200 16200]; [43 8578 7874 16200 16200 16200 16200 16200 16200 16200 16200 16200]; [44 11741 2686 16200 16200 16200 16200 16200 16200 16200 16200 16200]; [0 1022 1264 16200 16200 16200 16200 16200 16200 16200 16200 16200]; [1 12604 9965 16200 16200 16200 16200 16200 16200 16200 16200 16200]; [2 8217 2707 16200 16200 16200 16200 16200 16200 16200 16200 16200]; [3 3156 11793 16200 16200 16200 16200 16200 16200 16200 16200 16200]; [4 354 1514 16200 16200 16200 16200 16200 16200 16200 16200 16200]; [5 6978 14058 16200 16200 16200 16200 16200 16200 16200 16200 16200]; [6 7922 16079 16200 16200 16200 16200 16200 16200 16200 16200 16200]; [7 15087 12138 16200 16200 16200 16200 16200 16200 16200 16200 16200]; [8 5053 6470 16200 16200 16200 16200 16200 16200 16200 16200 16200]; [9 12687 14932 16200 16200 16200 16200 16200 16200 16200 16200 16200]; [10 15458 1763 16200 16200 16200 16200 16200 16200 16200 16200 16200]; [11 8121 1721 16200 16200 16200 16200 16200 16200 16200 16200 16200]; [12 12431 549 16200 16200 16200 16200 16200 16200 16200 16200 16200]; [13 4129 7091 16200 ...(+5412 chars)]]);, num_parity_bits=16200}
  bit_count : simulink/Logic and Bit Operations/Compare To Constant  relop===  const=359  OutDataTypeStr=boolean
  bit_counter1 : hdlsllib/Sources/HDL Counter  CountType=Count limited  CountInit=0  CountStep=1  CountMax=359  CountFromType=Initial value  CountFrom=0  CountResetPort=on  CountLoadPort=off  CountEnbPort=off  CountDirPort=off  CountDataType=Unsigned  CountWordLen=9  CountFracLen=0  CountSampTime=1
  q : Constant  Value=45  OutDataTypeStr=uint8  SampleTime=-1
  slot_counter : hdlsllib/Sources/HDL Counter  CountType=Count limited  CountInit=1  CountStep=1  CountMax=135  CountFromType=Initial value  CountFrom=1  CountResetPort=on  CountLoadPort=off  CountEnbPort=on  CountDirPort=off  CountDataType=Unsigned  CountWordLen=8  CountFracLen=0  CountSampTime=1
  addresses1 : Outport
  wires:
  addresses/1(addresses) -> addresses1/1
  bit_counter1/1 -> addresses/2(counter), bit_count/1
  bit_count/1 -> bit_counter1/1, slot_counter/2
  q/1 -> addresses/3(q_factor)
  rst/1 -> slot_counter/1
  slot_counter/1 -> addresses/1(slot)

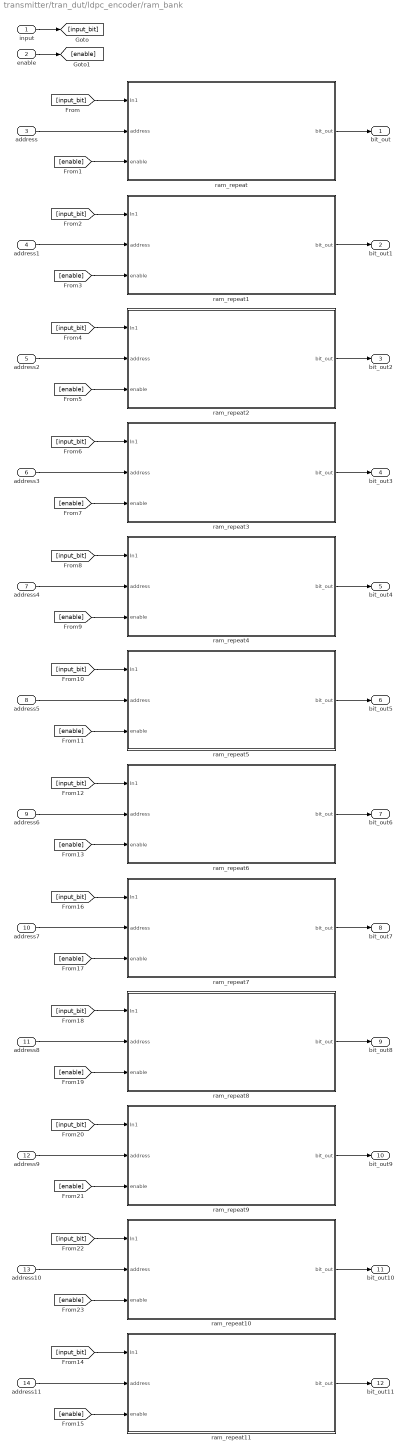
== system transmitter/tran_dut/ldpc_encoder/ram_bank ==
  input : Inport
  enable : Inport  Port=2
  address : Inport  Port=3
  address1 : Inport  Port=4
  address2 : Inport  Port=5
  address3 : Inport  Port=6
  address4 : Inport  Port=7
  address5 : Inport  Port=8
  address6 : Inport  Port=9
  address7 : Inport  Port=10
  address8 : Inport  Port=11
  address9 : Inport  Port=12
  address10 : Inport  Port=13
  address11 : Inport  Port=14
  ram_repeat : Subsystem
  ram_repeat1 : Subsystem
  ram_repeat10 : Subsystem
  ram_repeat11 : Subsystem
  ram_repeat2 : Subsystem
  ram_repeat3 : Subsystem
  ram_repeat4 : Subsystem
  ram_repeat5 : Subsystem
  ram_repeat6 : Subsystem
  ram_repeat7 : Subsystem
  ram_repeat8 : Subsystem
  ram_repeat9 : Subsystem
  bit_out : Outport
  bit_out1 : Outport  Port=2
  bit_out2 : Outport  Port=3
  bit_out3 : Outport  Port=4
  bit_out4 : Outport  Port=5
  bit_out5 : Outport  Port=6
  bit_out6 : Outport  Port=7
  bit_out7 : Outport  Port=8
  bit_out8 : Outport  Port=9
  bit_out9 : Outport  Port=10
  bit_out10 : Outport  Port=11
  bit_out11 : Outport  Port=12
  wires:
  ram_repeat/1(bit_out) -> bit_out/1
  address/1 -> ram_repeat/2(address)
  input/1 -> [input_bit]
  enable/1 -> [enable]
  [input_bit] -> ram_repeat/1(In1)
  [enable] -> ram_repeat/3(enable)
  [input_bit] -> ram_repeat1/1(In1)
  [enable] -> ram_repeat1/3(enable)
  ram_repeat1/1(bit_out) -> bit_out1/1
  address1/1 -> ram_repeat1/2(address)
  address3/1 -> ram_repeat3/2(address)
  ram_repeat2/1(bit_out) -> bit_out2/1
  ram_repeat3/1(bit_out) -> bit_out3/1
  [enable] -> ram_repeat3/3(enable)
  [input_bit] -> ram_repeat2/1(In1)
  [enable] -> ram_repeat2/3(enable)
  [input_bit] -> ram_repeat3/1(In1)
  address2/1 -> ram_repeat2/2(address)
  address5/1 -> ram_repeat5/2(address)
  ram_repeat4/1(bit_out) -> bit_out4/1
  ram_repeat5/1(bit_out) -> bit_out5/1
  [enable] -> ram_repeat5/3(enable)
  [input_bit] -> ram_repeat4/1(In1)
  [enable] -> ram_repeat4/3(enable)
  [input_bit] -> ram_repeat5/1(In1)
  address4/1 -> ram_repeat4/2(address)
  address6/1 -> ram_repeat6/2(address)
  [enable] -> ram_repeat9/3(enable)
  ram_repeat10/1(bit_out) -> bit_out10/1
  ram_repeat8/1(bit_out) -> bit_out8/1
  [input_bit] -> ram_repeat6/1(In1)
  [enable] -> ram_repeat10/3(enable)
  ram_repeat7/1(bit_out) -> bit_out7/1
  address10/1 -> ram_repeat10/2(address)
  [enable] -> ram_repeat6/3(enable)
  [input_bit] -> ram_repeat10/1(In1)
  address11/1 -> ram_repeat11/2(address)
  address9/1 -> ram_repeat9/2(address)
  address7/1 -> ram_repeat7/2(address)
  [enable] -> ram_repeat7/3(enable)
  ram_repeat9/1(bit_out) -> bit_out9/1
  [input_bit] -> ram_repeat8/1(In1)
  ram_repeat6/1(bit_out) -> bit_out6/1
  [input_bit] -> ram_repeat7/1(In1)
  [input_bit] -> ram_repeat11/1(In1)
  address8/1 -> ram_repeat8/2(address)
  [input_bit] -> ram_repeat9/1(In1)
  ram_repeat11/1(bit_out) -> bit_out11/1
  [enable] -> ram_repeat11/3(enable)
  [enable] -> ram_repeat8/3(enable)

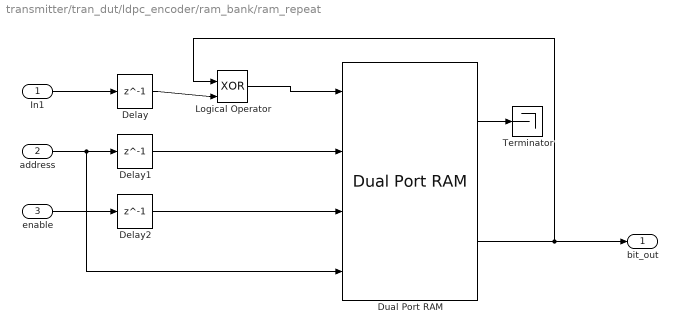
== system transmitter/tran_dut/ldpc_encoder/ram_bank/ram_repeat ==
  In1 : Inport
  address : Inport  Port=2
  enable : Inport  Port=3
  Delay : Delay  DelayLength=1
  Delay1 : Delay  DelayLength=1
  Delay2 : Delay  DelayLength=1
  Dual Port RAM : hdlsllib/HDL RAMs/Dual Port RAM  ram_size=14
      settings: SourceProductBaseCode=SL
  Logical Operator : Logic  Operator=XOR  IconShape=distinctive  AllPortsSameDT=off  OutDataTypeStr=boolean
  Terminator : Terminator
  bit_out : Outport
  wires:
  Dual Port RAM/1 -> Terminator/1
  Dual Port RAM/2 -> Logical Operator/1, bit_out/1
  Logical Operator/1 -> Dual Port RAM/1
  Delay/1 -> Logical Operator/2
  In1/1 -> Delay/1
  Delay1/1 -> Dual Port RAM/2
  address/1 -> Dual Port RAM/4, Delay1/1
  enable/1 -> Delay2/1
  Delay2/1 -> Dual Port RAM/3

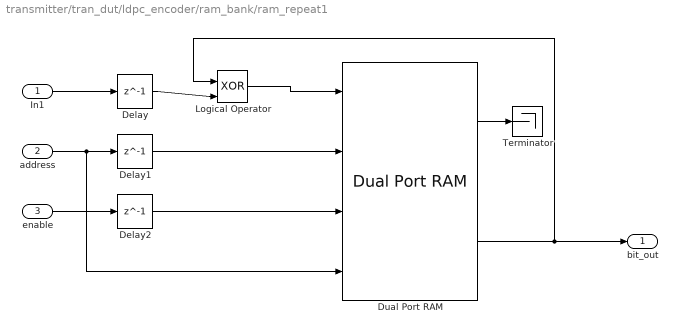
== system transmitter/tran_dut/ldpc_encoder/ram_bank/ram_repeat1 ==
  In1 : Inport
  address : Inport  Port=2
  enable : Inport  Port=3
  Delay : Delay  DelayLength=1
  Delay1 : Delay  DelayLength=1
  Delay2 : Delay  DelayLength=1
  Dual Port RAM : hdlsllib/HDL RAMs/Dual Port RAM  ram_size=14
      settings: SourceProductBaseCode=SL
  Logical Operator : Logic  Operator=XOR  IconShape=distinctive  AllPortsSameDT=off  OutDataTypeStr=boolean
  Terminator : Terminator
  bit_out : Outport
  wires:
  Dual Port RAM/1 -> Terminator/1
  Dual Port RAM/2 -> Logical Operator/1, bit_out/1
  Logical Operator/1 -> Dual Port RAM/1
  Delay/1 -> Logical Operator/2
  In1/1 -> Delay/1
  Delay1/1 -> Dual Port RAM/2
  address/1 -> Dual Port RAM/4, Delay1/1
  enable/1 -> Delay2/1
  Delay2/1 -> Dual Port RAM/3

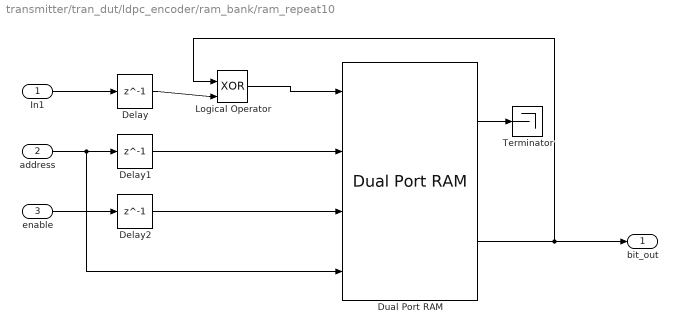
== system transmitter/tran_dut/ldpc_encoder/ram_bank/ram_repeat10 ==
  In1 : Inport
  address : Inport  Port=2
  enable : Inport  Port=3
  Delay : Delay  DelayLength=1
  Delay1 : Delay  DelayLength=1
  Delay2 : Delay  DelayLength=1
  Dual Port RAM : hdlsllib/HDL RAMs/Dual Port RAM  ram_size=14
      settings: SourceProductBaseCode=SL
  Logical Operator : Logic  Operator=XOR  IconShape=distinctive  AllPortsSameDT=off  OutDataTypeStr=boolean
  Terminator : Terminator
  bit_out : Outport
  wires:
  Dual Port RAM/1 -> Terminator/1
  Dual Port RAM/2 -> Logical Operator/1, bit_out/1
  Logical Operator/1 -> Dual Port RAM/1
  Delay/1 -> Logical Operator/2
  In1/1 -> Delay/1
  Delay1/1 -> Dual Port RAM/2
  address/1 -> Dual Port RAM/4, Delay1/1
  enable/1 -> Delay2/1
  Delay2/1 -> Dual Port RAM/3

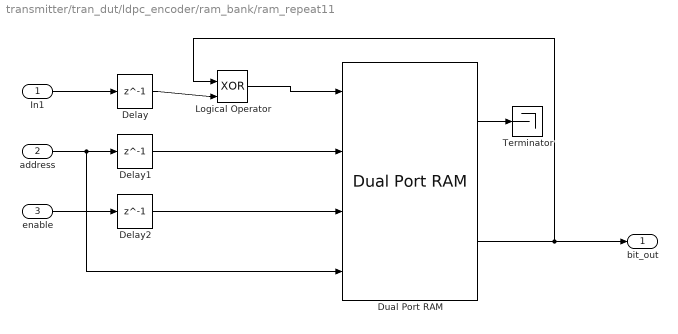
== system transmitter/tran_dut/ldpc_encoder/ram_bank/ram_repeat11 ==
  In1 : Inport
  address : Inport  Port=2
  enable : Inport  Port=3
  Delay : Delay  DelayLength=1
  Delay1 : Delay  DelayLength=1
  Delay2 : Delay  DelayLength=1
  Dual Port RAM : hdlsllib/HDL RAMs/Dual Port RAM  ram_size=14
      settings: SourceProductBaseCode=SL
  Logical Operator : Logic  Operator=XOR  IconShape=distinctive  AllPortsSameDT=off  OutDataTypeStr=boolean
  Terminator : Terminator
  bit_out : Outport
  wires:
  Dual Port RAM/1 -> Terminator/1
  Dual Port RAM/2 -> Logical Operator/1, bit_out/1
  Logical Operator/1 -> Dual Port RAM/1
  Delay/1 -> Logical Operator/2
  In1/1 -> Delay/1
  Delay1/1 -> Dual Port RAM/2
  address/1 -> Dual Port RAM/4, Delay1/1
  enable/1 -> Delay2/1
  Delay2/1 -> Dual Port RAM/3

== system transmitter/tran_dut/ldpc_encoder/ram_bank/ram_repeat2 ==
  In1 : Inport
  address : Inport  Port=2
  enable : Inport  Port=3
  Delay : Delay  DelayLength=1
  Delay1 : Delay  DelayLength=1
  Delay2 : Delay  DelayLength=1
  Dual Port RAM : hdlsllib/HDL RAMs/Dual Port RAM  ram_size=14
      settings: SourceProductBaseCode=SL
  Logical Operator : Logic  Operator=XOR  IconShape=distinctive  AllPortsSameDT=off  OutDataTypeStr=boolean
  Terminator : Terminator
  bit_out : Outport
  wires:
  Dual Port RAM/1 -> Terminator/1
  Dual Port RAM/2 -> Logical Operator/1, bit_out/1
  Logical Operator/1 -> Dual Port RAM/1
  Delay/1 -> Logical Operator/2
  In1/1 -> Delay/1
  Delay1/1 -> Dual Port RAM/2
  address/1 -> Dual Port RAM/4, Delay1/1
  enable/1 -> Delay2/1
  Delay2/1 -> Dual Port RAM/3

== system transmitter/tran_dut/ldpc_encoder/ram_bank/ram_repeat3 ==
  In1 : Inport
  address : Inport  Port=2
  enable : Inport  Port=3
  Delay : Delay  DelayLength=1
  Delay1 : Delay  DelayLength=1
  Delay2 : Delay  DelayLength=1
  Dual Port RAM : hdlsllib/HDL RAMs/Dual Port RAM  ram_size=14
      settings: SourceProductBaseCode=SL
  Logical Operator : Logic  Operator=XOR  IconShape=distinctive  AllPortsSameDT=off  OutDataTypeStr=boolean
  Terminator : Terminator
  bit_out : Outport
  wires:
  Dual Port RAM/1 -> Terminator/1
  Dual Port RAM/2 -> Logical Operator/1, bit_out/1
  Logical Operator/1 -> Dual Port RAM/1
  Delay/1 -> Logical Operator/2
  In1/1 -> Delay/1
  Delay1/1 -> Dual Port RAM/2
  address/1 -> Dual Port RAM/4, Delay1/1
  enable/1 -> Delay2/1
  Delay2/1 -> Dual Port RAM/3

== system transmitter/tran_dut/ldpc_encoder/ram_bank/ram_repeat4 ==
  In1 : Inport
  address : Inport  Port=2
  enable : Inport  Port=3
  Delay : Delay  DelayLength=1
  Delay1 : Delay  DelayLength=1
  Delay2 : Delay  DelayLength=1
  Dual Port RAM : hdlsllib/HDL RAMs/Dual Port RAM  ram_size=14
      settings: SourceProductBaseCode=SL
  Logical Operator : Logic  Operator=XOR  IconShape=distinctive  AllPortsSameDT=off  OutDataTypeStr=boolean
  Terminator : Terminator
  bit_out : Outport
  wires:
  Dual Port RAM/1 -> Terminator/1
  Dual Port RAM/2 -> Logical Operator/1, bit_out/1
  Logical Operator/1 -> Dual Port RAM/1
  Delay/1 -> Logical Operator/2
  In1/1 -> Delay/1
  Delay1/1 -> Dual Port RAM/2
  address/1 -> Dual Port RAM/4, Delay1/1
  enable/1 -> Delay2/1
  Delay2/1 -> Dual Port RAM/3

== system transmitter/tran_dut/ldpc_encoder/ram_bank/ram_repeat5 ==
  In1 : Inport
  address : Inport  Port=2
  enable : Inport  Port=3
  Delay : Delay  DelayLength=1
  Delay1 : Delay  DelayLength=1
  Delay2 : Delay  DelayLength=1
  Dual Port RAM : hdlsllib/HDL RAMs/Dual Port RAM  ram_size=14
      settings: SourceProductBaseCode=SL
  Logical Operator : Logic  Operator=XOR  IconShape=distinctive  AllPortsSameDT=off  OutDataTypeStr=boolean
  Terminator : Terminator
  bit_out : Outport
  wires:
  Dual Port RAM/1 -> Terminator/1
  Dual Port RAM/2 -> Logical Operator/1, bit_out/1
  Logical Operator/1 -> Dual Port RAM/1
  Delay/1 -> Logical Operator/2
  In1/1 -> Delay/1
  Delay1/1 -> Dual Port RAM/2
  address/1 -> Dual Port RAM/4, Delay1/1
  enable/1 -> Delay2/1
  Delay2/1 -> Dual Port RAM/3

== system transmitter/tran_dut/ldpc_encoder/ram_bank/ram_repeat6 ==
  In1 : Inport
  address : Inport  Port=2
  enable : Inport  Port=3
  Delay : Delay  DelayLength=1
  Delay1 : Delay  DelayLength=1
  Delay2 : Delay  DelayLength=1
  Dual Port RAM : hdlsllib/HDL RAMs/Dual Port RAM  ram_size=14
      settings: SourceProductBaseCode=SL
  Logical Operator : Logic  Operator=XOR  IconShape=distinctive  AllPortsSameDT=off  OutDataTypeStr=boolean
  Terminator : Terminator
  bit_out : Outport
  wires:
  Dual Port RAM/1 -> Terminator/1
  Dual Port RAM/2 -> Logical Operator/1, bit_out/1
  Logical Operator/1 -> Dual Port RAM/1
  Delay/1 -> Logical Operator/2
  In1/1 -> Delay/1
  Delay1/1 -> Dual Port RAM/2
  address/1 -> Dual Port RAM/4, Delay1/1
  enable/1 -> Delay2/1
  Delay2/1 -> Dual Port RAM/3

== system transmitter/tran_dut/ldpc_encoder/ram_bank/ram_repeat7 ==
  In1 : Inport
  address : Inport  Port=2
  enable : Inport  Port=3
  Delay : Delay  DelayLength=1
  Delay1 : Delay  DelayLength=1
  Delay2 : Delay  DelayLength=1
  Dual Port RAM : hdlsllib/HDL RAMs/Dual Port RAM  ram_size=14
      settings: SourceProductBaseCode=SL
  Logical Operator : Logic  Operator=XOR  IconShape=distinctive  AllPortsSameDT=off  OutDataTypeStr=boolean
  Terminator : Terminator
  bit_out : Outport
  wires:
  Dual Port RAM/1 -> Terminator/1
  Dual Port RAM/2 -> Logical Operator/1, bit_out/1
  Logical Operator/1 -> Dual Port RAM/1
  Delay/1 -> Logical Operator/2
  In1/1 -> Delay/1
  Delay1/1 -> Dual Port RAM/2
  address/1 -> Dual Port RAM/4, Delay1/1
  enable/1 -> Delay2/1
  Delay2/1 -> Dual Port RAM/3

== system transmitter/tran_dut/ldpc_encoder/ram_bank/ram_repeat8 ==
  In1 : Inport
  address : Inport  Port=2
  enable : Inport  Port=3
  Delay : Delay  DelayLength=1
  Delay1 : Delay  DelayLength=1
  Delay2 : Delay  DelayLength=1
  Dual Port RAM : hdlsllib/HDL RAMs/Dual Port RAM  ram_size=14
      settings: SourceProductBaseCode=SL
  Logical Operator : Logic  Operator=XOR  IconShape=distinctive  AllPortsSameDT=off  OutDataTypeStr=boolean
  Terminator : Terminator
  bit_out : Outport
  wires:
  Dual Port RAM/1 -> Terminator/1
  Dual Port RAM/2 -> Logical Operator/1, bit_out/1
  Logical Operator/1 -> Dual Port RAM/1
  Delay/1 -> Logical Operator/2
  In1/1 -> Delay/1
  Delay1/1 -> Dual Port RAM/2
  address/1 -> Dual Port RAM/4, Delay1/1
  enable/1 -> Delay2/1
  Delay2/1 -> Dual Port RAM/3

== system transmitter/tran_dut/ldpc_encoder/ram_bank/ram_repeat9 ==
  In1 : Inport
  address : Inport  Port=2
  enable : Inport  Port=3
  Delay : Delay  DelayLength=1
  Delay1 : Delay  DelayLength=1
  Delay2 : Delay  DelayLength=1
  Dual Port RAM : hdlsllib/HDL RAMs/Dual Port RAM  ram_size=14
      settings: SourceProductBaseCode=SL
  Logical Operator : Logic  Operator=XOR  IconShape=distinctive  AllPortsSameDT=off  OutDataTypeStr=boolean
  Terminator : Terminator
  bit_out : Outport
  wires:
  Dual Port RAM/1 -> Terminator/1
  Dual Port RAM/2 -> Logical Operator/1, bit_out/1
  Logical Operator/1 -> Dual Port RAM/1
  Delay/1 -> Logical Operator/2
  In1/1 -> Delay/1
  Delay1/1 -> Dual Port RAM/2
  address/1 -> Dual Port RAM/4, Delay1/1
  enable/1 -> Delay2/1
  Delay2/1 -> Dual Port RAM/3

== matlab function transmitter/tran_dut/bit_mapping/angle_selector ==
  settings: fimath=fimath('RoundingMethod', 'Floor','OverflowAction', 'Wrap','ProductMode', 'FullPrecision', 'SumMode', 'FullPrecision')
  data: input input; phase output
function phase = phase_selector(input)
%#codegen
% Receives a bit sequence and returns the angle in radians of the
% corresponding 8-psk constellation symbol. Gray encoding is used as stated
% in the DVB-S2 standard.
    tmp = 0; % Start at phase 0
    if(input == 1)
        tmp=0;
    elseif(input == 0)
        tmp=45;
    elseif(input == 4)
        tmp=90;
    elseif(input == 6)
        tmp=135;
    elseif(input == 2)
        tmp=180;
    elseif(input == 3)
        tmp=225;
    elseif(input == 7)
        tmp=270;
    elseif(input == 5)
        tmp=315;
    end
    % 9 bits necessary to represent 360 degrees.
    phase = fi(tmp, 0, 23, 14, hdlfimath);
